simulink model "Fig351"  (R2014b)
settings: Solver=ode3  StartTime=0.0  StopTime=10.002  FixedStep=2e-6  RelTol=1e-5
libraries: dsparch4 x2, commchan3 x1, dspstat3 x1, commrandsrc2 x1
settings Model: Creator=Dennis Silage  LastModifiedBy=Silage
settings DataIOCC: SignalLoggingSaveFormat=ModelDataLogs
settings OptimizationCC: ExpressionDepthLimit=2147483647  InitFltsAndDblsToZero=on
settings DebuggingCC: UnderspecifiedInitializationDetection=Classic  MergeDetectMultiDrivingBlocksExec=none  SolverPrmCheckMsg=none  FcnCallInpInsideContextMsg=UseLocalSettings  StateNameClashWarn=warning
settings GRTTargetCC: CombineOutputUpdateFcns=off  GRTInterface=on

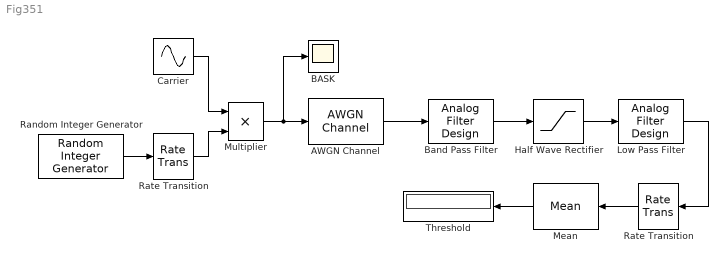
== system Fig351 ==
  AWGN Channel : commchan3/AWGN Channel  InputProcessing=Inherited (this choice will be removed - see release notes)  seed=randseed  noiseMode="Signal to noise ratio  (Eb/No)"  EbNodB=80  EsNodB=10  SNRdB=12  bitsPerSym=1  Ps=12.5  Tsym=1e-3  variance=0
  BASK : Scope
      settings: YMin=-6  YMax=6
  Band Pass Filter : dsparch4/Analog Filter Design  method=Butterworth  filttype=Bandpass  N=9  Wlo=38000*pi  Whi=42000*pi  Rp=2  Rs=40
  Carrier : Sin  Amplitude=5  Frequency=40000*pi  SampleTime=2e-6
  Half Wave Rectifier : Saturate  UpperLimit=2000  LowerLimit=0
  Low Pass Filter : dsparch4/Analog Filter Design  method=Butterworth  filttype=Lowpass  N=9  Wlo=4000*pi  Whi=46000*pi  Rp=2  Rs=40
  Mean : dspstat3/Mean  run=on  reset_popup=None  InputProcessing=Inherited (this choice will be removed - see release notes)  directionMode=Each column  dimension=1  treatSBRowAsCol=on  roiEnable=off  roiType=Rectangles  roiPortion=Entire ROI  roiOutput=Individual statistics for each ROI  roiFlag=off  outputDataTypeStr=Inherit: Same as accumulator  outputLastDataTypeStr=Inherit: Same as accumulator  outputMin=[]  outputMax=[]  roundingMode=Floor  overflowMode=off
  "Multiplier " : Product  RndMeth=Zero
  Random Integer Generator : commrandsrc2/Random Integer Generator  mul=2  seed=randseed  Ts=1e-3  frameBased=off  sampPerFrame=50  orient=on  outDataType=double
  "Rate Transition " : RateTransition  OutPortSampleTime=2e-6
  Rate Transition : RateTransition  OutPortSampleTime=2e-6
  Threshold : Display
  wires:
  Random Integer Generator/1 -> Rate Transition/1
  "Multiplier "/1 -> AWGN Channel/1, BASK/1
  Carrier/1 -> "Multiplier "/1
  Rate Transition/1 -> "Multiplier "/2
  Band Pass Filter/1 -> Half Wave Rectifier/1
  Half Wave Rectifier/1 -> Low Pass Filter/1
  Mean/1 -> Threshold/1
  AWGN Channel/1 -> Band Pass Filter/1
  "Rate Transition "/1 -> Mean/1
  Low Pass Filter/1 -> "Rate Transition "/1
